simulink model "модель манипулятора"  (R2018a)
settings: Solver=VariableStepAuto  StartTime=0.0  StopTime=10  RelTol=1e-3
libraries: simulink x8
settings Model: Creator=user  LastModifiedBy=user

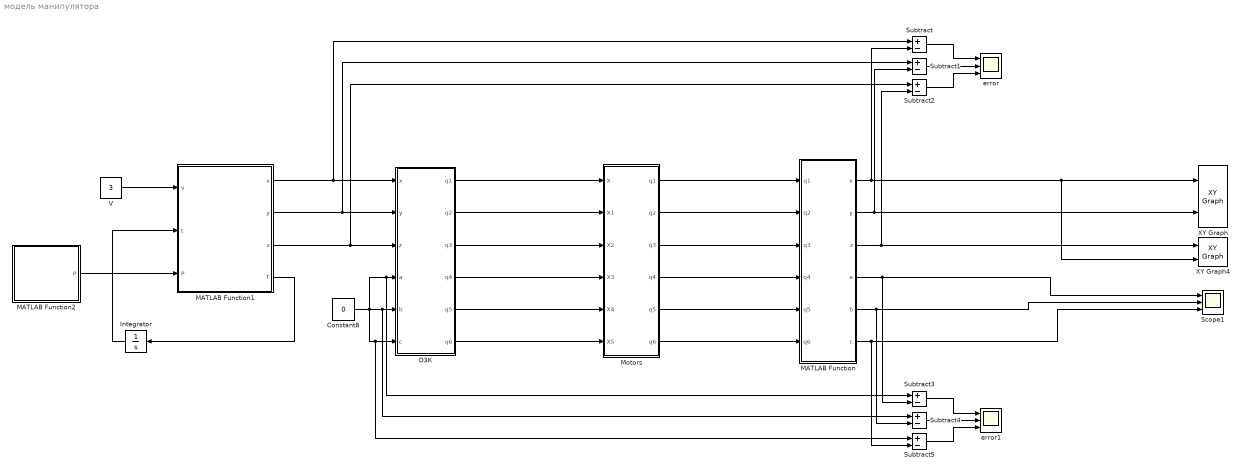
== system модель манипулятора ==
  Constant8 : Constant  Value=0
  Integrator : Integrator
  MATLAB Function : MATLAB Function  TreatAsAtomicUnit=on
  MATLAB Function1 : MATLAB Function  TreatAsAtomicUnit=on
  MATLAB Function2 : MATLAB Function  TreatAsAtomicUnit=on
  Motors : Subsystem
  Scope1 : Scope  NumInputPorts=3
  Subtract{,1..5} (6 alike) : Sum  Inputs=+-
  V : Constant  Value=3
  XY Graph : simulink/Sinks/XY Graph  xmin=-2  xmax=2  ymin=-2  ymax=2  st=-1
  XY Graph4 : simulink/Sinks/XY Graph  xmin=-2  xmax=2  ymin=-2  ymax=2  st=-1
  error : Scope  NumInputPorts=3
  error1 : Scope  NumInputPorts=3
  ОЗК : MATLAB Function  TreatAsAtomicUnit=on
  wires:
  Constant8/1 -> Subtract3/1, ОЗК/4(a), Subtract5/1, ОЗК/6(c), Subtract4/1, ОЗК/5(b)
  MATLAB Function/1(x) -> Subtract/2, XY Graph4/2, XY Graph/1
  MATLAB Function/2(y) -> Subtract1/2, XY Graph/2
  MATLAB Function/3(z) -> Subtract2/2, XY Graph4/1
  MATLAB Function/4(a) -> Subtract3/2, Scope1/1
  MATLAB Function/5(b) -> Subtract4/2, Scope1/2
  MATLAB Function/6(c) -> Subtract5/2, Scope1/3
  ОЗК/3(q3) -> Motors/3(X2)
  ОЗК/4(q4) -> Motors/4(X3)
  ОЗК/5(q5) -> Motors/5(X4)
  ОЗК/6(q6) -> Motors/6(X5)
  ОЗК/1(q1) -> Motors/1(X)
  ОЗК/2(q2) -> Motors/2(X1)
  Motors/3(q3) -> MATLAB Function/3(q3)
  Motors/2(q2) -> MATLAB Function/2(q2)
  Motors/1(q1) -> MATLAB Function/1(q1)
  Motors/4(q4) -> MATLAB Function/4(q4)
  Motors/5(q5) -> MATLAB Function/5(q5)
  Motors/6(q6) -> MATLAB Function/6(q6)
  MATLAB Function1/4(T) -> Integrator/1
  Integrator/1 -> MATLAB Function1/2(t)
  V/1 -> MATLAB Function1/1(v)
  MATLAB Function1/3(z) -> Subtract2/1, ОЗК/3(z)
  MATLAB Function1/2(y) -> Subtract1/1, ОЗК/2(y)
  MATLAB Function1/1(x) -> Subtract/1, ОЗК/1(x)
  MATLAB Function2/1(P) -> MATLAB Function1/3(P)
  Subtract/1 -> error/1
  Subtract1/1 -> error/2
  Subtract2/1 -> error/3
  Subtract5/1 -> error1/3
  Subtract4/1 -> error1/2
  Subtract3/1 -> error1/1

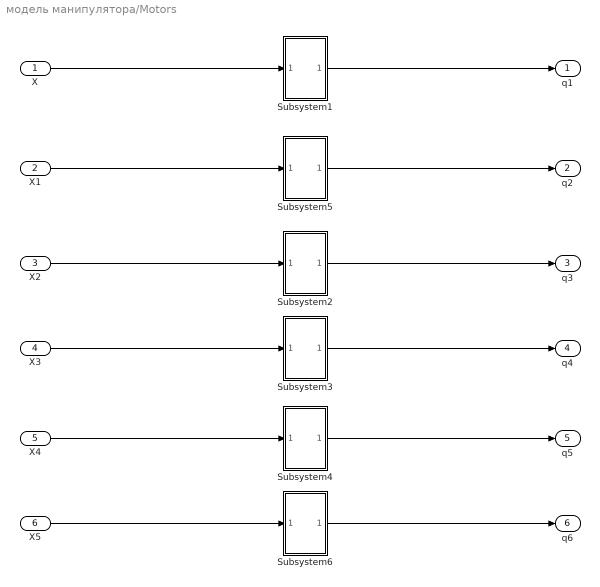
== system модель манипулятора/Motors ==
  X : Inport
  X1 : Inport  Port=2
  X2 : Inport  Port=3
  X3 : Inport  Port=4
  X4 : Inport  Port=5
  X5 : Inport  Port=6
  Subsystem1 : Subsystem
  Subsystem2 : Subsystem
  Subsystem3 : Subsystem
  Subsystem4 : Subsystem
  Subsystem5 : Subsystem
  Subsystem6 : Subsystem
  q1 : Outport
  q2 : Outport  Port=2
  q3 : Outport  Port=3
  q4 : Outport  Port=4
  q5 : Outport  Port=5
  q6 : Outport  Port=6
  wires:
  X/1 -> Subsystem1/1(In2)
  Subsystem1/1(Out2) -> q1/1
  Subsystem5/1(Out2) -> q2/1
  X1/1 -> Subsystem5/1(In2)
  X2/1 -> Subsystem2/1(In2)
  Subsystem2/1(Out2) -> q3/1
  Subsystem3/1(Out2) -> q4/1
  X3/1 -> Subsystem3/1(In2)
  X4/1 -> Subsystem4/1(In2)
  Subsystem4/1(Out2) -> q5/1
  Subsystem6/1(Out2) -> q6/1
  X5/1 -> Subsystem6/1(In2)

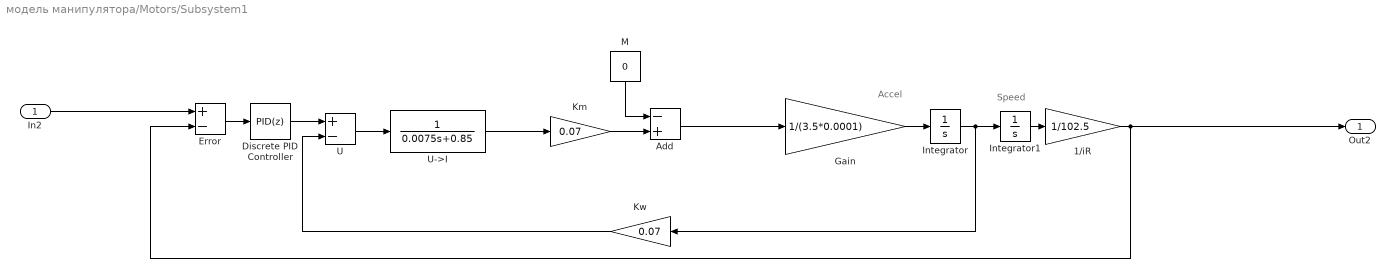
== system модель манипулятора/Motors/Subsystem1 ==
  note: Accel
  note: Speed
  In2 : Inport
  1/iR : Gain  Gain=1/102.5
  Add : Sum  Inputs=-+
  Discrete PID Controller : simulink/Continuous/PID Controller  Controller=PID  TimeDomain=Discrete-time  SampleTime=-1  IntegratorMethod=Forward Euler  FilterMethod=Forward Euler  Form=Parallel  UseFilter=on  ControllerParametersSource=internal  P=34.35  I=4.909  D=2.866  N=5.543  InitialConditionSource=internal  InitialConditionForIntegrator=0  InitialConditionForFilter=0  ExternalReset=none  LimitOutput=off  UpperSaturationLimit=inf  LowerSaturationLimit=-inf  LinearizeAsGain=off  AntiWindupMode=none  Kb=1  TrackingMode=off  Kt=1  PParamMin=[]  PParamMax=[]  IParamMin=[]  IParamMax=[]  DParamMin=[]  DParamMax=[]  NParamMin=[]  NParamMax=[]  KbParamMin=[]  KbParamMax=[]  KtParamMin=[]  KtParamMax=[]  POutMin=[]  POutMax=[]  IOutMin=[]  IOutMax=[]  DOutMin=[]  DOutMax=[]  NOutMin=[]  NOutMax=[]  KbOutMin=[]  KbOutMax=[]  KtOutMin=[]  KtOutMax=[]  IntegratorOutMin=[]  IntegratorOutMax=[]  FilterOutMin=[]  FilterOutMax=[]  SumOutMin=[]  SumOutMax=[]  SumI1OutMin=[]  SumI1OutMax=[]  SumI2OutMin=[]  SumI2OutMax=[]  SumI3OutMin=[]  SumI3OutMax=[]  SumDOutMin=[]  SumDOutMax=[]  SaturationOutMin=[]  SaturationOutMax=[]  IntegratorContinuousStateAttributes=''  IntegratorStateMustResolveToSignalObject=off  IntegratorRTWStateStorageClass=Auto  FilterContinuousStateAttributes=''  FilterStateMustResolveToSignalObject=off  FilterRTWStateStorageClass=Auto  DifferentiatorICPrevScaledInput=0  DifferentiatorOutMin=[]  DifferentiatorOutMax=[]  FilterDiffOutCoefMin=[]  FilterDiffOutCoefMax=[]  SumDenOutMin=[]  SumDenOutMax=[]  SumNumOutMin=[]  SumNumOutMax=[]  ReciprocalOutMin=[]  ReciprocalOutMax=[]  DivideOutMin=[]  DivideOutMax=[]  TunerSelectOption=Transfer Function Based (PID Tuner App)
  "Error " : Sum  Inputs=+-
  Gain : Gain  Gain=1/(3.5*0.0001)
  Integrator : Integrator
  Integrator1 : Integrator  InitialCondition=1.1618*102.5
  Km : Gain  Gain=0.07
  Kw : Gain  Gain=0.07
  "M " : Constant  Value=0
  U : Sum  Inputs=+-
  U->I : TransferFcn  Denominator=[0.0075 0.85]
  Out2 : Outport
  wires:
  Km/1 -> Add/2
  Add/1 -> Gain/1
  Discrete PID Controller/1 -> U/1
  Kw/1 -> U/2
  1/iR/1 -> Out2/1, "Error "/2
  "Error "/1 -> Discrete PID Controller/1
  Integrator/1 -> Integrator1/1, Kw/1
  "M "/1 -> Add/1
  U->I/1 -> Km/1
  Gain/1 -> Integrator/1
  U/1 -> U->I/1
  Integrator1/1 -> 1/iR/1
  In2/1 -> "Error "/1

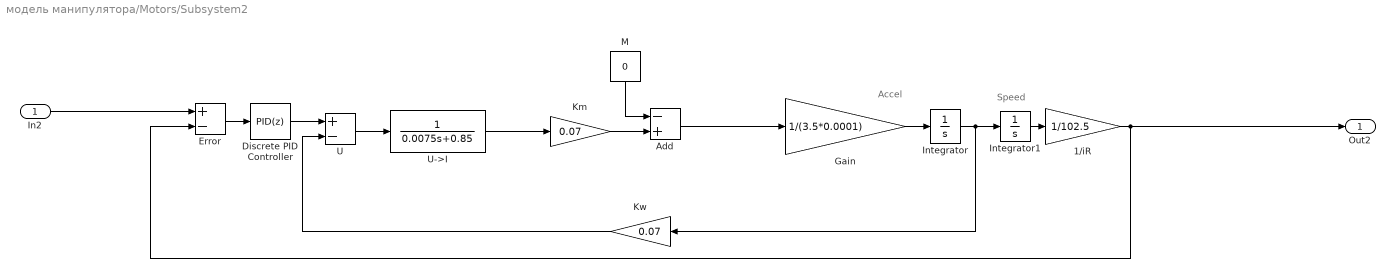
== system модель манипулятора/Motors/Subsystem2 ==
  note: Speed
  note: Accel
  In2 : Inport
  1/iR : Gain  Gain=1/102.5
  Add : Sum  Inputs=-+
  Discrete PID Controller : simulink/Continuous/PID Controller  Controller=PID  TimeDomain=Discrete-time  SampleTime=-1  IntegratorMethod=Forward Euler  FilterMethod=Forward Euler  Form=Parallel  UseFilter=on  ControllerParametersSource=internal  P=34.35  I=4.909  D=2.866  N=5.543  InitialConditionSource=internal  InitialConditionForIntegrator=0  InitialConditionForFilter=0  ExternalReset=none  LimitOutput=off  UpperSaturationLimit=inf  LowerSaturationLimit=-inf  LinearizeAsGain=off  AntiWindupMode=none  Kb=1  TrackingMode=off  Kt=1  PParamMin=[]  PParamMax=[]  IParamMin=[]  IParamMax=[]  DParamMin=[]  DParamMax=[]  NParamMin=[]  NParamMax=[]  KbParamMin=[]  KbParamMax=[]  KtParamMin=[]  KtParamMax=[]  POutMin=[]  POutMax=[]  IOutMin=[]  IOutMax=[]  DOutMin=[]  DOutMax=[]  NOutMin=[]  NOutMax=[]  KbOutMin=[]  KbOutMax=[]  KtOutMin=[]  KtOutMax=[]  IntegratorOutMin=[]  IntegratorOutMax=[]  FilterOutMin=[]  FilterOutMax=[]  SumOutMin=[]  SumOutMax=[]  SumI1OutMin=[]  SumI1OutMax=[]  SumI2OutMin=[]  SumI2OutMax=[]  SumI3OutMin=[]  SumI3OutMax=[]  SumDOutMin=[]  SumDOutMax=[]  SaturationOutMin=[]  SaturationOutMax=[]  IntegratorContinuousStateAttributes=''  IntegratorStateMustResolveToSignalObject=off  IntegratorRTWStateStorageClass=Auto  FilterContinuousStateAttributes=''  FilterStateMustResolveToSignalObject=off  FilterRTWStateStorageClass=Auto  DifferentiatorICPrevScaledInput=0  DifferentiatorOutMin=[]  DifferentiatorOutMax=[]  FilterDiffOutCoefMin=[]  FilterDiffOutCoefMax=[]  SumDenOutMin=[]  SumDenOutMax=[]  SumNumOutMin=[]  SumNumOutMax=[]  ReciprocalOutMin=[]  ReciprocalOutMax=[]  DivideOutMin=[]  DivideOutMax=[]  TunerSelectOption=Transfer Function Based (PID Tuner App)
  "Error " : Sum  Inputs=+-
  Gain : Gain  Gain=1/(3.5*0.0001)
  Integrator : Integrator
  Integrator1 : Integrator  InitialCondition=1.1618*102.5
  Km : Gain  Gain=0.07
  Kw : Gain  Gain=0.07
  "M " : Constant  Value=0
  U : Sum  Inputs=+-
  U->I : TransferFcn  Denominator=[0.0075 0.85]
  Out2 : Outport
  wires:
  In2/1 -> "Error "/1
  Integrator1/1 -> 1/iR/1
  U/1 -> U->I/1
  Gain/1 -> Integrator/1
  U->I/1 -> Km/1
  "M "/1 -> Add/1
  Integrator/1 -> Kw/1, Integrator1/1
  "Error "/1 -> Discrete PID Controller/1
  1/iR/1 -> "Error "/2, Out2/1
  Kw/1 -> U/2
  Discrete PID Controller/1 -> U/1
  Add/1 -> Gain/1
  Km/1 -> Add/2

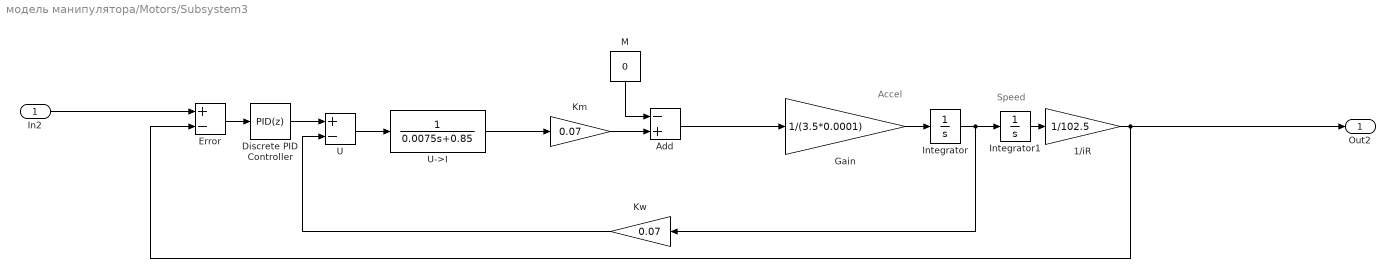
== system модель манипулятора/Motors/Subsystem3 ==
  note: Accel
  note: Speed
  In2 : Inport
  1/iR : Gain  Gain=1/102.5
  Add : Sum  Inputs=-+
  Discrete PID Controller : simulink/Continuous/PID Controller  Controller=PID  TimeDomain=Discrete-time  SampleTime=-1  IntegratorMethod=Forward Euler  FilterMethod=Forward Euler  Form=Parallel  UseFilter=on  ControllerParametersSource=internal  P=34.35  I=4.909  D=2.866  N=5.543  InitialConditionSource=internal  InitialConditionForIntegrator=0  InitialConditionForFilter=0  ExternalReset=none  LimitOutput=off  UpperSaturationLimit=inf  LowerSaturationLimit=-inf  LinearizeAsGain=off  AntiWindupMode=none  Kb=1  TrackingMode=off  Kt=1  PParamMin=[]  PParamMax=[]  IParamMin=[]  IParamMax=[]  DParamMin=[]  DParamMax=[]  NParamMin=[]  NParamMax=[]  KbParamMin=[]  KbParamMax=[]  KtParamMin=[]  KtParamMax=[]  POutMin=[]  POutMax=[]  IOutMin=[]  IOutMax=[]  DOutMin=[]  DOutMax=[]  NOutMin=[]  NOutMax=[]  KbOutMin=[]  KbOutMax=[]  KtOutMin=[]  KtOutMax=[]  IntegratorOutMin=[]  IntegratorOutMax=[]  FilterOutMin=[]  FilterOutMax=[]  SumOutMin=[]  SumOutMax=[]  SumI1OutMin=[]  SumI1OutMax=[]  SumI2OutMin=[]  SumI2OutMax=[]  SumI3OutMin=[]  SumI3OutMax=[]  SumDOutMin=[]  SumDOutMax=[]  SaturationOutMin=[]  SaturationOutMax=[]  IntegratorContinuousStateAttributes=''  IntegratorStateMustResolveToSignalObject=off  IntegratorRTWStateStorageClass=Auto  FilterContinuousStateAttributes=''  FilterStateMustResolveToSignalObject=off  FilterRTWStateStorageClass=Auto  DifferentiatorICPrevScaledInput=0  DifferentiatorOutMin=[]  DifferentiatorOutMax=[]  FilterDiffOutCoefMin=[]  FilterDiffOutCoefMax=[]  SumDenOutMin=[]  SumDenOutMax=[]  SumNumOutMin=[]  SumNumOutMax=[]  ReciprocalOutMin=[]  ReciprocalOutMax=[]  DivideOutMin=[]  DivideOutMax=[]  TunerSelectOption=Transfer Function Based (PID Tuner App)
  "Error " : Sum  Inputs=+-
  Gain : Gain  Gain=1/(3.5*0.0001)
  Integrator : Integrator
  Integrator1 : Integrator  InitialCondition=1.1618*102.5
  Km : Gain  Gain=0.07
  Kw : Gain  Gain=0.07
  "M " : Constant  Value=0
  U : Sum  Inputs=+-
  U->I : TransferFcn  Denominator=[0.0075 0.85]
  Out2 : Outport
  wires:
  Km/1 -> Add/2
  Add/1 -> Gain/1
  Discrete PID Controller/1 -> U/1
  Kw/1 -> U/2
  1/iR/1 -> Out2/1, "Error "/2
  "Error "/1 -> Discrete PID Controller/1
  Integrator/1 -> Integrator1/1, Kw/1
  "M "/1 -> Add/1
  U->I/1 -> Km/1
  Gain/1 -> Integrator/1
  U/1 -> U->I/1
  Integrator1/1 -> 1/iR/1
  In2/1 -> "Error "/1

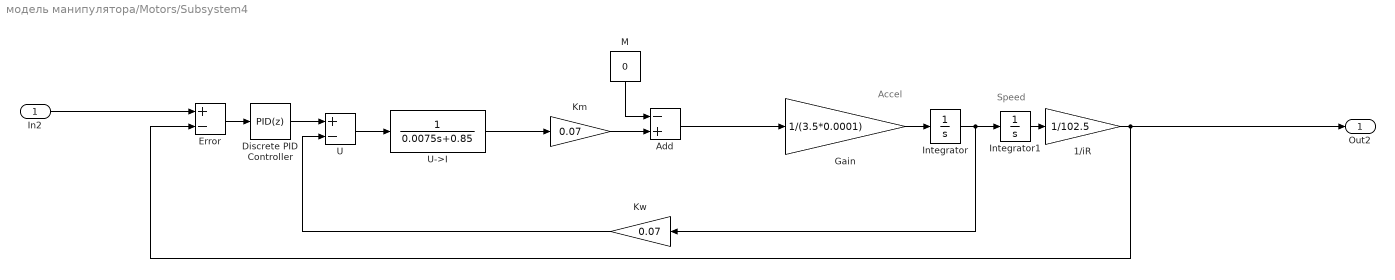
== system модель манипулятора/Motors/Subsystem4 ==
  note: Speed
  note: Accel
  In2 : Inport
  1/iR : Gain  Gain=1/102.5
  Add : Sum  Inputs=-+
  Discrete PID Controller : simulink/Continuous/PID Controller  Controller=PID  TimeDomain=Discrete-time  SampleTime=-1  IntegratorMethod=Forward Euler  FilterMethod=Forward Euler  Form=Parallel  UseFilter=on  ControllerParametersSource=internal  P=34.35  I=4.909  D=2.866  N=5.543  InitialConditionSource=internal  InitialConditionForIntegrator=0  InitialConditionForFilter=0  ExternalReset=none  LimitOutput=off  UpperSaturationLimit=inf  LowerSaturationLimit=-inf  LinearizeAsGain=off  AntiWindupMode=none  Kb=1  TrackingMode=off  Kt=1  PParamMin=[]  PParamMax=[]  IParamMin=[]  IParamMax=[]  DParamMin=[]  DParamMax=[]  NParamMin=[]  NParamMax=[]  KbParamMin=[]  KbParamMax=[]  KtParamMin=[]  KtParamMax=[]  POutMin=[]  POutMax=[]  IOutMin=[]  IOutMax=[]  DOutMin=[]  DOutMax=[]  NOutMin=[]  NOutMax=[]  KbOutMin=[]  KbOutMax=[]  KtOutMin=[]  KtOutMax=[]  IntegratorOutMin=[]  IntegratorOutMax=[]  FilterOutMin=[]  FilterOutMax=[]  SumOutMin=[]  SumOutMax=[]  SumI1OutMin=[]  SumI1OutMax=[]  SumI2OutMin=[]  SumI2OutMax=[]  SumI3OutMin=[]  SumI3OutMax=[]  SumDOutMin=[]  SumDOutMax=[]  SaturationOutMin=[]  SaturationOutMax=[]  IntegratorContinuousStateAttributes=''  IntegratorStateMustResolveToSignalObject=off  IntegratorRTWStateStorageClass=Auto  FilterContinuousStateAttributes=''  FilterStateMustResolveToSignalObject=off  FilterRTWStateStorageClass=Auto  DifferentiatorICPrevScaledInput=0  DifferentiatorOutMin=[]  DifferentiatorOutMax=[]  FilterDiffOutCoefMin=[]  FilterDiffOutCoefMax=[]  SumDenOutMin=[]  SumDenOutMax=[]  SumNumOutMin=[]  SumNumOutMax=[]  ReciprocalOutMin=[]  ReciprocalOutMax=[]  DivideOutMin=[]  DivideOutMax=[]  TunerSelectOption=Transfer Function Based (PID Tuner App)
  "Error " : Sum  Inputs=+-
  Gain : Gain  Gain=1/(3.5*0.0001)
  Integrator : Integrator
  Integrator1 : Integrator  InitialCondition=1.1618*102.5
  Km : Gain  Gain=0.07
  Kw : Gain  Gain=0.07
  "M " : Constant  Value=0
  U : Sum  Inputs=+-
  U->I : TransferFcn  Denominator=[0.0075 0.85]
  Out2 : Outport
  wires:
  In2/1 -> "Error "/1
  Integrator1/1 -> 1/iR/1
  U/1 -> U->I/1
  Gain/1 -> Integrator/1
  U->I/1 -> Km/1
  "M "/1 -> Add/1
  Integrator/1 -> Kw/1, Integrator1/1
  "Error "/1 -> Discrete PID Controller/1
  1/iR/1 -> "Error "/2, Out2/1
  Kw/1 -> U/2
  Discrete PID Controller/1 -> U/1
  Add/1 -> Gain/1
  Km/1 -> Add/2

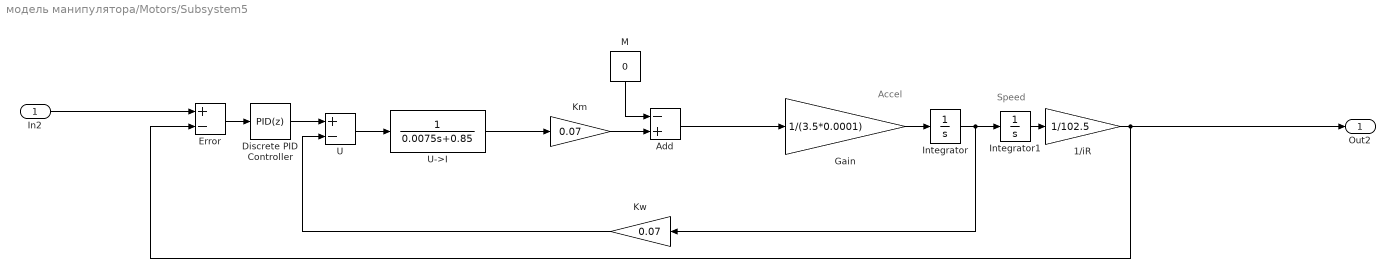
== system модель манипулятора/Motors/Subsystem5 ==
  note: Speed
  note: Accel
  In2 : Inport
  1/iR : Gain  Gain=1/102.5
  Add : Sum  Inputs=-+
  Discrete PID Controller : simulink/Continuous/PID Controller  Controller=PID  TimeDomain=Discrete-time  SampleTime=-1  IntegratorMethod=Forward Euler  FilterMethod=Forward Euler  Form=Parallel  UseFilter=on  ControllerParametersSource=internal  P=34.35  I=4.909  D=2.866  N=5.543  InitialConditionSource=internal  InitialConditionForIntegrator=0  InitialConditionForFilter=0  ExternalReset=none  LimitOutput=off  UpperSaturationLimit=inf  LowerSaturationLimit=-inf  LinearizeAsGain=off  AntiWindupMode=none  Kb=1  TrackingMode=off  Kt=1  PParamMin=[]  PParamMax=[]  IParamMin=[]  IParamMax=[]  DParamMin=[]  DParamMax=[]  NParamMin=[]  NParamMax=[]  KbParamMin=[]  KbParamMax=[]  KtParamMin=[]  KtParamMax=[]  POutMin=[]  POutMax=[]  IOutMin=[]  IOutMax=[]  DOutMin=[]  DOutMax=[]  NOutMin=[]  NOutMax=[]  KbOutMin=[]  KbOutMax=[]  KtOutMin=[]  KtOutMax=[]  IntegratorOutMin=[]  IntegratorOutMax=[]  FilterOutMin=[]  FilterOutMax=[]  SumOutMin=[]  SumOutMax=[]  SumI1OutMin=[]  SumI1OutMax=[]  SumI2OutMin=[]  SumI2OutMax=[]  SumI3OutMin=[]  SumI3OutMax=[]  SumDOutMin=[]  SumDOutMax=[]  SaturationOutMin=[]  SaturationOutMax=[]  IntegratorContinuousStateAttributes=''  IntegratorStateMustResolveToSignalObject=off  IntegratorRTWStateStorageClass=Auto  FilterContinuousStateAttributes=''  FilterStateMustResolveToSignalObject=off  FilterRTWStateStorageClass=Auto  DifferentiatorICPrevScaledInput=0  DifferentiatorOutMin=[]  DifferentiatorOutMax=[]  FilterDiffOutCoefMin=[]  FilterDiffOutCoefMax=[]  SumDenOutMin=[]  SumDenOutMax=[]  SumNumOutMin=[]  SumNumOutMax=[]  ReciprocalOutMin=[]  ReciprocalOutMax=[]  DivideOutMin=[]  DivideOutMax=[]  TunerSelectOption=Transfer Function Based (PID Tuner App)
  "Error " : Sum  Inputs=+-
  Gain : Gain  Gain=1/(3.5*0.0001)
  Integrator : Integrator
  Integrator1 : Integrator  InitialCondition=1.1618*102.5
  Km : Gain  Gain=0.07
  Kw : Gain  Gain=0.07
  "M " : Constant  Value=0
  U : Sum  Inputs=+-
  U->I : TransferFcn  Denominator=[0.0075 0.85]
  Out2 : Outport
  wires:
  In2/1 -> "Error "/1
  Integrator1/1 -> 1/iR/1
  U/1 -> U->I/1
  Gain/1 -> Integrator/1
  U->I/1 -> Km/1
  "M "/1 -> Add/1
  Integrator/1 -> Kw/1, Integrator1/1
  "Error "/1 -> Discrete PID Controller/1
  1/iR/1 -> "Error "/2, Out2/1
  Kw/1 -> U/2
  Discrete PID Controller/1 -> U/1
  Add/1 -> Gain/1
  Km/1 -> Add/2

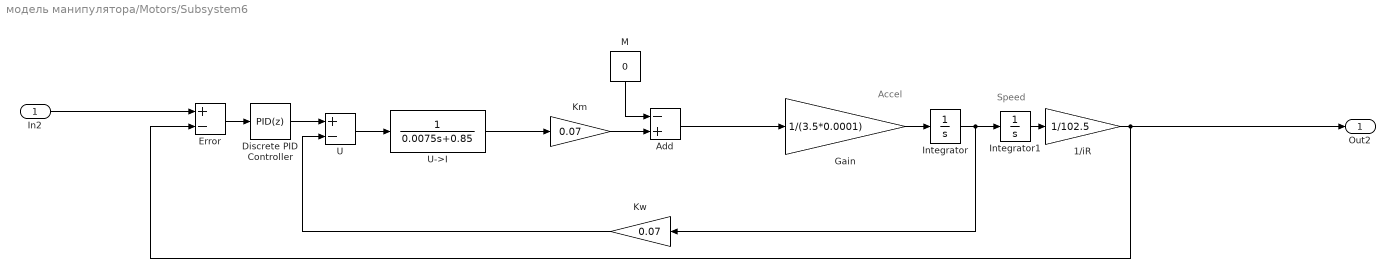
== system модель манипулятора/Motors/Subsystem6 ==
  note: Accel
  note: Speed
  In2 : Inport
  1/iR : Gain  Gain=1/102.5
  Add : Sum  Inputs=-+
  Discrete PID Controller : simulink/Continuous/PID Controller  Controller=PID  TimeDomain=Discrete-time  SampleTime=-1  IntegratorMethod=Forward Euler  FilterMethod=Forward Euler  Form=Parallel  UseFilter=on  ControllerParametersSource=internal  P=34.35  I=4.909  D=2.866  N=5.543  InitialConditionSource=internal  InitialConditionForIntegrator=0  InitialConditionForFilter=0  ExternalReset=none  LimitOutput=off  UpperSaturationLimit=inf  LowerSaturationLimit=-inf  LinearizeAsGain=off  AntiWindupMode=none  Kb=1  TrackingMode=off  Kt=1  PParamMin=[]  PParamMax=[]  IParamMin=[]  IParamMax=[]  DParamMin=[]  DParamMax=[]  NParamMin=[]  NParamMax=[]  KbParamMin=[]  KbParamMax=[]  KtParamMin=[]  KtParamMax=[]  POutMin=[]  POutMax=[]  IOutMin=[]  IOutMax=[]  DOutMin=[]  DOutMax=[]  NOutMin=[]  NOutMax=[]  KbOutMin=[]  KbOutMax=[]  KtOutMin=[]  KtOutMax=[]  IntegratorOutMin=[]  IntegratorOutMax=[]  FilterOutMin=[]  FilterOutMax=[]  SumOutMin=[]  SumOutMax=[]  SumI1OutMin=[]  SumI1OutMax=[]  SumI2OutMin=[]  SumI2OutMax=[]  SumI3OutMin=[]  SumI3OutMax=[]  SumDOutMin=[]  SumDOutMax=[]  SaturationOutMin=[]  SaturationOutMax=[]  IntegratorContinuousStateAttributes=''  IntegratorStateMustResolveToSignalObject=off  IntegratorRTWStateStorageClass=Auto  FilterContinuousStateAttributes=''  FilterStateMustResolveToSignalObject=off  FilterRTWStateStorageClass=Auto  DifferentiatorICPrevScaledInput=0  DifferentiatorOutMin=[]  DifferentiatorOutMax=[]  FilterDiffOutCoefMin=[]  FilterDiffOutCoefMax=[]  SumDenOutMin=[]  SumDenOutMax=[]  SumNumOutMin=[]  SumNumOutMax=[]  ReciprocalOutMin=[]  ReciprocalOutMax=[]  DivideOutMin=[]  DivideOutMax=[]  TunerSelectOption=Transfer Function Based (PID Tuner App)
  "Error " : Sum  Inputs=+-
  Gain : Gain  Gain=1/(3.5*0.0001)
  Integrator : Integrator
  Integrator1 : Integrator  InitialCondition=1.1618*102.5
  Km : Gain  Gain=0.07
  Kw : Gain  Gain=0.07
  "M " : Constant  Value=0
  U : Sum  Inputs=+-
  U->I : TransferFcn  Denominator=[0.0075 0.85]
  Out2 : Outport
  wires:
  Km/1 -> Add/2
  Add/1 -> Gain/1
  Discrete PID Controller/1 -> U/1
  Kw/1 -> U/2
  1/iR/1 -> Out2/1, "Error "/2
  "Error "/1 -> Discrete PID Controller/1
  Integrator/1 -> Integrator1/1, Kw/1
  "M "/1 -> Add/1
  U->I/1 -> Km/1
  Gain/1 -> Integrator/1
  U/1 -> U->I/1
  Integrator1/1 -> 1/iR/1
  In2/1 -> "Error "/1

== matlab function модель манипулятора/ОЗК ==
  data: x input; q1 output; y input; z input; q2 output; q3 output; a input; b input; c input; q4 output; q5 output; q6 output
function[q1,q2,q3,q4,q5,q6] = IK(x,y,z,a,b,c)
%This function is used for inverse kinematics calculations.

%link lenghts in mm


d1=0.4865;
d2=0.150;
d3=0.475;
d4=0.600;
d6=0.065;

alpha = [-pi/2, 0, -pi/2, pi/2, -pi/2, 0];
% a = [d2 d3 0 0 0 0];
% d = [d1 0 0 d4 0 d6];

%%%%%%%%%%%%%%%%%Inverse kinematics%%%%%%%%%%%%%%%%%

R06= [cos(a)*cos(b), cos(a)*sin(c)*sin(b)-sin(a)*cos(c), cos(a)*sin(b)*cos(c)+sin(a)*sin(c);
      sin(a)*cos(b), sin(a)*sin(b)*sin(c)+cos(a)*cos(c), sin(a)*sin(b)*cos(c)-cos(a)*sin(c);
      - sin(b),      cos(b)*sin(c),                      cos(b)*cos(c)];
% R06=[cos(a)*cos(c)*cos(b)-sin(a)*sin(c),-cos(a)*sin(c)*cos(b)-sin(a)*cos(c),cos(a)*sin(b);
%     sin(a)*cos(c)*cos(b)-cos(a)*sin(c),-sin(a)*cos(b)*sin(c)+cos(a)*cos(c),sin(a)*sin(b);
%     -sin(b)*cos(c),sin(b)*sin(c),cos(b)];

p06=[x y z];
p04=p06-transpose(d6*R06*[0;0;1]);
% xc = x - d6*R(1,3);
% yc = y - d6*R(2,3);
% zc = z - d6*R(3,3);
xc=p04(1);
yc=p04(2);
zc=p04(3);

% r = sqrt(xc^2 + yc^2);

%Inverse kinematic equations for position
theta1 = atan2(yc,xc);

r = (xc^2 + yc^2)^(1/2);
D = ((r - d2)^2 + (zc - d1)^2 - d3^2 - d4^2)/(2*d3*d4);

theta3_dash = atan2((-(1 - D^2)^(1/2)), D);
theta3 = abs(theta3_dash) - (90*pi/180);

theta2_dash = (atan2( zc-d1, r-d2) - atan2(d4*sind(theta3_dash*180/pi),d3+d4*cosd(theta3_dash*180/pi))) ;
theta2 = (90*pi/180) - theta2_dash;

theta5 = atan2(sqrt(1-(sin(theta1)*R06(1,3)- cos(theta1)*R06(2,3))^2),sin(theta1)*R06(1,3) - cos(theta1)*R06(2,3)) -pi;
theta4 = atan2(-cos(theta1)*sin(theta2+theta3)*R06(1,3)-sin(theta1)*sin(theta2+theta3)*R06(2,3)+cos(theta2+theta3)*R06(3,3),cos(theta1)*cos(theta2+theta3)*R06(1,3)+sin(theta1)*cos(theta2+theta3)*R06(2,3)+sin(theta2+theta3)*R06(3,3));
theta6= atan2(sin(theta1)*R06(1,2)-cos(theta1)*R06(2,2),-sin(theta1)*R06(1,1)+cos(theta1)*R06(2,1));

%Converting angles to degrees, because angles passed as arguments to the
%function forwardKinematics() have to be in degrees.
q1 = theta1 * 180 / pi;
q2 = theta2 * 180 / pi;
q3 = theta3 * 180 / pi;
q4 = theta4 * 180 / pi;
q5 = theta5 * 180 / pi;
q6 = theta6 * 180 / pi;

end

== matlab function модель манипулятора/MATLAB Function ==
  data: q1 input; x output; y output; z output; a output; b output; c output; q2 input; q3 input; q4 input; q5 input; q6 input
function [x,y,z,a,b,c] = DK(q1,q2,q3,q4,q5,q6)

%   i       Link twist     Link Length     Link Offset    Joint Angle    
%--------------------------------------------------------------------------
%   1        -90              d2             d1                 theta1*     
%   2         0               d3              0               theta2 - 90*  
%   3        -90               0              0                 theta3*     
%   4         90               0             d4                 theta4*     
%   5        -90               0              0                 theta5*     
%   6         0                0             d5                 theta6*     


d1=0.4865;
d2=0.150;
d3=0.475;
d4=0.600;
d6=0.065;
sc=10000;

% q1=q1/180*pi;
% q2=q2/180*pi;
% q3=q3/180*pi;
% q4=q4/180*pi;
% q5=q5/180*pi;
% q6=q6/180*pi;

T01 = make_tfMatrix(d2, -90, q1 ,d1);  
T12 = make_tfMatrix(d3,  0, q2 - 90,   0);%-162.835/sc);
T23 = make_tfMatrix(0, -90,      q3    ,0);% 162.835/sc);
T34 = make_tfMatrix(0,  90,      q4    , d4); 
T45 = make_tfMatrix(0, -90,      q5    , 0);
T56 = make_tfMatrix(0,   0,      q6    , d6);

T06=T01*T12*T23*T34*T45*T56;
T03=T01*T12*T23;

x=T06(1,4);
y=T06(2,4);
z=T06(3,4);

R06=T06(1:3,1:3);
R03=T03(1:3,1:3);
R36=R06*transpose(R03);
if R36(3,3)==1
    a=0;
    c=0;
    b=atan2(R06(2,1),R06(1,1));
elseif R36(3,3)==-1
     a=0;
     c=0;
     b=atan2(-R36(1,2),-R36(1,1));
else
    a=atan2(R36(2,3),R36(1,3));
    b=atan2(R36(3,2),-R36(3,1));
    c=atan2(sqrt(1-R36(3,3)^2),R36(3,3));
end

function [ transformation_matrix ] = make_tfMatrix( a, alpha, th, d )


transformation_matrix = [cosd(th),   -sind(th)*cosd(alpha),      sind(th)*sind(alpha),      a*cosd(th);
                         sind(th),    cosd(th)*cosd(alpha),     -cosd(th)*sind(alpha),      a*sind(th);
                              0  ,          sind(alpha)   ,          cosd(alpha)     ,           d    ;
                              0  ,             0          ,               0          ,            1   ];

end
    
end

== matlab function модель манипулятора/MATLAB Function1 ==
  data: x output; v input; y output; t input; P input; z output; T output
function [x,y,z,T] = TargetPosition(v,t,P)

  i=2;
  for k = 1:1:length(P)-3
    if (t>k)
     i = k+2;
    end
  end
  t = t - i+2;

    Ak=zeros(1,3);
    Bk=zeros(1,3);
    Ck=zeros(1,3);
    Dk=zeros(1,3);
    F=zeros(1,3);
    S=zeros(1,3);
    
    for j=1:3
    Ak(j)=(-P(j,i-1)+3*P(j,i)-3*P(j,i+1)+P(j,i+2))/6;
    Bk(j)=(3*P(j,i-1)-6*P(j,i)+3*P(j,i+1))/6;
    Ck(j)=(-3*P(j,i-1)+3*P(j,i+1))/6;
    Dk(j)=(P(j,i-1)+4*P(j,i)+P(j,i+1))/6;
    F(j)=3*Ak(j)*t^2+2*Bk(j)*t+Ck(j);
    S(j)=Ak(j)*t^3+Bk(j)*t^2+Ck(j)*t+Dk(j);
    end
    T=v/sqrt(F(1)^2+F(2)^2+F(3)^2);
    
    x=S(1);
    y=S(2);
    z=S(3);



end

== matlab function модель манипулятора/MATLAB Function2 ==
  data: P output
function P = fcn()
 Px   = [10 12.5 15 15 15 12.5 10 7.5 5 5 5 7.5 10 12.5 15 15 15 12.5 10 7.5 5 5 5 7.5];
 Py   = [5 5 7.5 10 12.5 15 15 15 12.5 10 7.5 5 5 5 7.5 10 12.5 15 15 15 12.5 10 7.5 5]; 
 Pz   = [6 6 6 6 6 6 6 6 6 6 6 6 6 6 6 6 6 6 6 6 6 6 6 6];
P=[Px;Py;Pz];
end
